simulink model "videocurvefitraspi"  (R2022a)
settings: Solver=FixedStepAuto  StartTime=0.0  StopTime=10.0  RelTol=1e-3  EnableMultiTasking=on
libraries: visionconversions x2, raspberrypiAVlib x2, visiontextngfix x1
settings Model: Creator=akuno  LastModifiedBy=akuno
settings SolverCC: PositivePriorityOrder=on
settings OptimizationCC: EnhancedBackFolding=on  PassReuseOutputArgsAs=Individual arguments  ZeroExternalMemoryAtStartup=off  ZeroInternalMemoryAtStartup=off  MaxStackSize=64  OptimizeBlockOrder=speed  DifferentSizesBufferReuse=on  OptimizationCustomize=off  EfficientTunableParamExpr=on
settings DebuggingCC: ParameterTunabilityLossMsg=error
settings HardwareCC: ProdBitPerPointer=32  ProdBitPerSizeT=32  ProdBitPerPtrDiffT=32  ProdLargestAtomicInteger=Long  ProdLargestAtomicFloat=Double  ProdWordSize=32  ProdLongLongMode=on  ProdHWDeviceType=ARM Compatible->ARM Cortex
settings RTWCC: SystemTargetFile=ert.tlc  HardwareBoard=Raspberry Pi  TLCOptions="-aInlineSetEventsForThisBaseRateFcn=TLC_FALSE -aSuppressMultiTaskScheduler=TLC_FALSE  -aRateBasedStepFcn=0"  TemplateMakefile=ert_default_tmf  Toolchain=GNU GCC Embedded Linux  BuildConfiguration=Faster Runs
settings CodeAppCC: ForceParamTrailComments=on  IgnoreCustomStorageClasses=off  OperatorAnnotations=on  SimulinkDataObjDesc=on  SFDataObjDesc=on  InsertBlockDesc=on
settings ERTTargetCC: SupportVariableSizeSignals=on  ExtModeTransport=2  ExtModeStaticAlloc=on  ExtModeMexFile=ext_xcp  ExtModeIntrfLevel=Level2 - Open

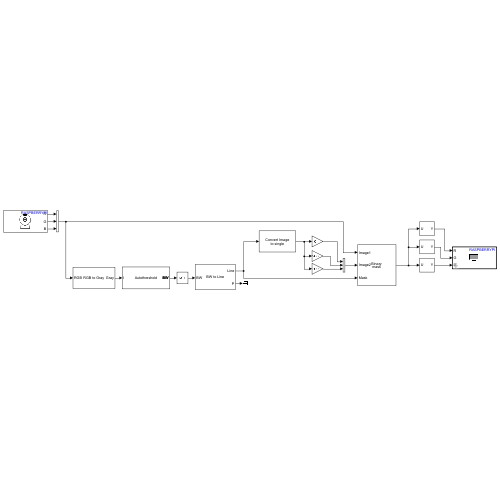
[thumbnail: Simulink's stored preview of the top-level diagram]
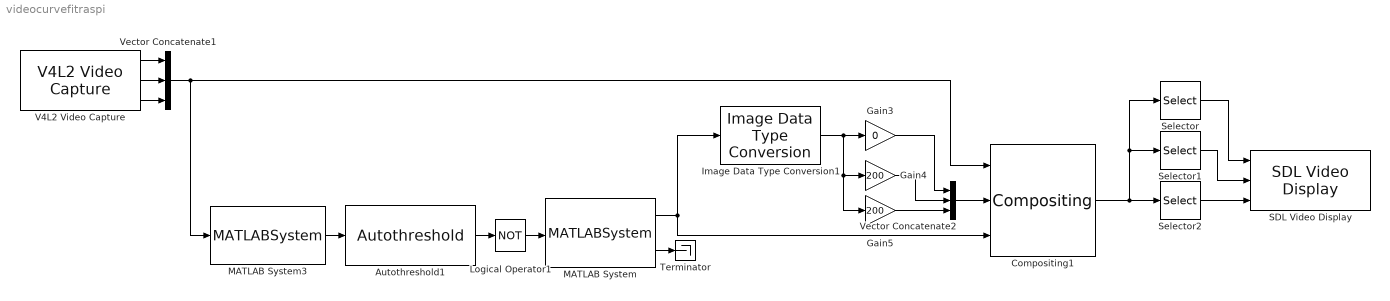
== system videocurvefitraspi ==
  Autothreshold1 : visionconversions/Autothreshold  operator=>  threshOut=off  effMetricOut=off  userDefinedRange=off  umin=0  umax=255  outOfRngOpt=Ignore  scaleThreshold=off  scaleFactor=1  roundingMode=Floor  overflowMode=off  P1Mode=Specify word length  P1WordLength=32  P1FracLength=30  P2Mode=Specify word length  P2WordLength=32  P2FracLength=22  P3Mode=Specify word length  P3WordLength=32  P3FracLength=14  P4Mode=Binary point scaling  P4WordLength=32  P4FracLength=15  Q1Mode=Specify word length  Q1WordLength=32  Q1FracLength=16  EMMode=Specify word length  EMWordLength=16  EMFracLength=14
      settings: SourceProductBaseCode=VP
  Compositing1 : visiontextngfix/Compositing  operation=Binary mask  bFacSrc=Specify via dialog  bFactor=0.5  mFacSrc=Input port  mFactor=1  source=Specify via dialog  coordinates=[1 1]  roundingMode=Floor  overflowMode=off  prodOutputMode=Binary point scaling  prodOutputWordLength=32  prodOutputFracLength=10
      settings: SourceProductBaseCode=VP
  Gain3 : Gain  Gain=0  ParamDataTypeStr=uint8  OutDataTypeStr=uint8
  Gain4 : Gain  Gain=200  ParamDataTypeStr=uint8  OutDataTypeStr=uint8
  Gain5 : Gain  Gain=200  ParamDataTypeStr=uint8  OutDataTypeStr=uint8
  Image Data Type Conversion1 : visionconversions/Image Data Type Conversion  outDT=single  isSigned=on  wordLen=16  numFracBits=0
      settings: SourceProductBaseCode=VP
  Logical Operator1 : Logic  Operator=NOT  AllPortsSameDT=off  OutDataTypeStr=boolean
  MATLAB System : MATLABSystem  System=CurveDetectionSystem  Degree=3  SimulateUsing=Code generation
      mask Type: CurveDetectionSystem
      mask Display:
      | disp('BW to Line');
      | port_label('input',1,'BW');
      | port_label('output',1,'Line');
      | port_label('output',2,'P');
  MATLAB System3 : MATLABSystem  System=Rgb2GraySystem  SimulateUsing=Code generation
      mask Type: Rgb2GraySystem
      mask Display:
      | disp('RGB to Gray');
      | port_label('input',1,'RGB');
      | port_label('output',1,'Gray');
  SDL Video Display : raspberrypiAVlib/SDL Video Display  title=SDL Video Display  pixelFormat=RGB  pixelOrder=Planar  rowMajor=on  blockPlatform=Raspberry Pi
      settings: SourceProductBaseCode=SC_BEAGLEBONE_BLUE,EMBEDDEDLINUX,NVIDIA,RASPPIIO
  Selector : Selector  NumberOfDimensions=3  InputPortWidth=3  IndexOptions=Select all,Select all,Index vector (dialog)  Indices=[1 3],1,1  OutputSizes=1,1,1
  Selector1 : Selector  NumberOfDimensions=3  InputPortWidth=3  IndexOptions=Select all,Select all,Index vector (dialog)  Indices=[1 3],1,2  OutputSizes=1,1,1
  Selector2 : Selector  NumberOfDimensions=3  InputPortWidth=3  IndexOptions=Select all,Select all,Index vector (dialog)  Indices=[1 3],1,3  OutputSizes=1,1,1
  Terminator : Terminator
  V4L2 Video Capture : raspberrypiAVlib/V4L2 Video Capture  DeviceName=/dev/video0  Resolution=160x120  CustomResolution=[ 320, 240 ]  PixelFormat=RGB  SampleTime=0.1  pixelOrder=planar  simOutput=Colorbars  imSizeSelection=320x240  imSize=[640, 480]  roi=[0, 0, 640, 480]  m_devName='/dev/video0'  blockPlatform=LINUX  HorizontalFlip=off  VerticalFlip=off  Brightness=0.5  Saturation=0.5  Contrast=0.5  Sharpness=0.5  CameraPan=0  CameraTilt=0  CameraZoom=0.5  EnableManualFocus=on  ManualFocus=0.5
      settings: SourceProductBaseCode=RASPPI
  Vector Concatenate1 : Concatenate  NumInputs=3  Mode=Multidimensional array  ConcatenateDimension=3
  Vector Concatenate2 : Concatenate  NumInputs=3  Mode=Multidimensional array  ConcatenateDimension=3
  wires:
  Compositing1/1 -> Selector/1, Selector1/1, Selector2/1
  V4L2 Video Capture/1 -> Vector Concatenate1/1
  V4L2 Video Capture/2 -> Vector Concatenate1/2
  V4L2 Video Capture/3 -> Vector Concatenate1/3
  Selector/1 -> SDL Video Display/1
  Selector1/1 -> SDL Video Display/2
  Selector2/1 -> SDL Video Display/3
  Gain4/1 -> Vector Concatenate2/2
  Vector Concatenate2/1 -> Compositing1/2
  MATLAB System3/1 -> Autothreshold1/1
  Autothreshold1/1 -> Logical Operator1/1
  MATLAB System/1 -> Compositing1/3, Image Data Type Conversion1/1
  Gain3/1 -> Vector Concatenate2/1
  Gain5/1 -> Vector Concatenate2/3
  Logical Operator1/1 -> MATLAB System/1
  Vector Concatenate1/1 -> MATLAB System3/1, Compositing1/1
  Image Data Type Conversion1/1 -> Gain4/1, Gain5/1, Gain3/1
  MATLAB System/2 -> Terminator/1
